simulink model "ac3_lat"  (Simulink 5.0)
settings: Solver=ode45  StartTime=0.0  StopTime=1000  RelTol=1e-3
values from neighbouring files (symbols this model uses):
  Dwash = [tau_w 1]    [ac3.m]
  JDa = [tau_a 1]    [ac3.m]
  JDr = [tau_r 1]    [ac3.m]
  JNa = [0 1]    [ac3.m]
  JNr = [0 1]    [ac3.m]
  Kphi = -30    [ac3.m]
  Nwash = [tau_w 0]    [ac3.m]
  rgain = (U0/g/tau_h)    (= 2.0039075773)    [ac3.m]
  theta0 = 0    [ac3.m]    (also in altit_simul.m; lecture4.m)
  U0 = 235.9    [ac3.m]    (also in altit_simul.m; lecture4.m = 774; newr.m)
libraries: aerolibanim x1, cstblocks x1
settings Model: LastModifiedBy=jonathan How

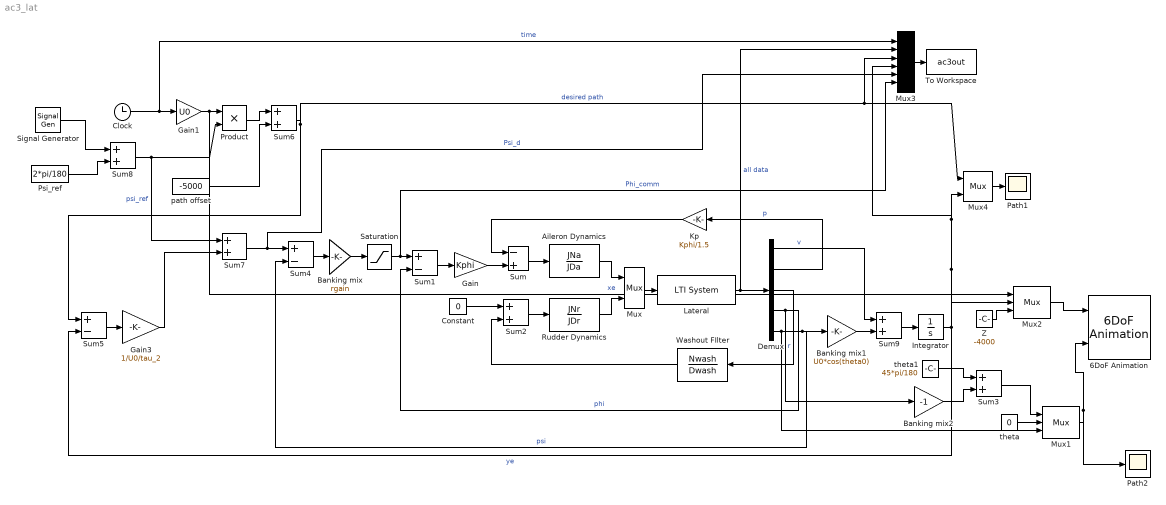
== system ac3_lat ==
  6DoF Animation : aerolibanim/6DoF Animation  u1=[0 4000 -6000 2000 -5000 -3000]  u2=0.1  u3=10  u4=[4000 0 -5000]  u5=Fly alongside  u6=[-100 0 -10]  u7=10  u8=on
  Aileron Dynamics : TransferFcn  Numerator=JNa  Denominator=JDa
  Banking mix : Gain  Gain=rgain  SaturateOnIntegerOverflow=on
  Banking mix1 : Gain  Gain=U0*cos(theta0)  SaturateOnIntegerOverflow=on
  Banking mix2 : Gain  Gain=-1  SaturateOnIntegerOverflow=on
  Clock : Clock
      settings: Decimation=10
  Constant : Constant  Value=0
  Demux : Demux  Outputs=5
  Gain : Gain  Gain=Kphi  SaturateOnIntegerOverflow=on
  Gain1 : Gain  Gain=U0  SaturateOnIntegerOverflow=on
  Gain3 : Gain  Gain=1/U0/tau_2  SaturateOnIntegerOverflow=on
  Integrator : Integrator
  Kp : Gain  Orientation=left  Gain=Kphi/1.5  SaturateOnIntegerOverflow=on
  Lateral : cstblocks/LTI System  sys=syslat2  IC=0
  Mux : Mux  Inputs=2
  Mux1 : Mux  Inputs=3
  Mux2 : Mux  Inputs=3
  Mux3 : Mux  Inputs=6
  Mux4 : Mux  Inputs=2
      settings: DisplayOption=signals
  Path1 : Scope
      settings: TimeRange=1000  YMin=-8000  YMax=9000
  Path2 : Scope
      settings: TimeRange=1000  YMin=-0.5  YMax=1.4
  Product : Product  SaturateOnIntegerOverflow=on  InputSameDT=on
  Psi_ref : Constant  Value=2*pi/180
  Rudder Dynamics : TransferFcn  Numerator=JNr  Denominator=JDr
  Saturation : Saturate  UpperLimit=30*pi/180  LowerLimit=-30*pi/180
  Signal Generator : SignalGenerator  WaveForm=square  Amplitude=3*pi/180  Frequency=.015  Units=rad/sec
  Sum : Sum  Inputs=-+  SaturateOnIntegerOverflow=on  InputSameDT=on
  Sum1 : Sum  Inputs=+-  SaturateOnIntegerOverflow=on  InputSameDT=on
  Sum{2..3,6..9} (6 alike) : Sum  SaturateOnIntegerOverflow=on  InputSameDT=on
  Sum4 : Sum  Inputs=+-  SaturateOnIntegerOverflow=on  InputSameDT=on
  Sum5 : Sum  Inputs=+-  SaturateOnIntegerOverflow=on  InputSameDT=on
  To Workspace : ToWorkspace  VariableName=ac3out  SampleTime=-1  SaveFormat=Array
  Washout FIlter : TransferFcn  Orientation=left  Numerator=Nwash  Denominator=Dwash
  Z : Constant  Value=-4000
  path offset : Constant  Value=-5000
  theta : Constant  Value=0
  theta1 : Constant  Value=45*pi/180
  wires:
  Aileron Dynamics/1 -> Mux/1
  Rudder Dynamics/1 -> Mux/2
  Mux/1 -> Lateral/1
  Lateral/1 -> Demux/1, Mux3/2  "all data"
  Demux/3 -> Washout FIlter/1  "r"
  Constant/1 -> Sum2/1
  Sum2/1 -> Rudder Dynamics/1
  Washout FIlter/1 -> Sum2/2
  Demux/2 -> Kp/1  "p"
  Kp/1 -> Sum/1
  Sum/1 -> Aileron Dynamics/1
  Demux/4 -> Sum1/2, Banking mix2/1  "phi"
  Sum1/1 -> Gain/1
  Demux/1 -> Sum9/1  "v"
  Demux/5 -> Sum4/2, Banking mix1/1, Mux1/3  "psi"
  Gain/1 -> Sum/2
  Sum4/1 -> Banking mix/1
  Banking mix/1 -> Saturation/1
  Product/1 -> Sum6/1
  Psi_ref/1 -> Sum8/2
  Signal Generator/1 -> Sum8/1
  Clock/1 -> Gain1/1, Mux3/1  "time"
  Gain1/1 -> Product/1, Mux2/1  "xe"
  path offset/1 -> Sum6/2
  Sum6/1 -> Sum5/1, Mux4/1, Mux3/3  "desired path"
  Sum8/1 -> Sum7/1, Product/2  "psi_ref"
  Sum7/1 -> Sum4/1, Mux3/5  "Psi_d"
  Sum5/1 -> Gain3/1
  Gain3/1 -> Sum7/2
  Banking mix1/1 -> Sum9/2
  Sum9/1 -> Integrator/1
  Integrator/1 -> Sum5/2, Mux4/2, Mux3/4, Mux2/2  "ye"
  Mux4/1 -> Path1/1
  Mux3/1 -> To Workspace/1
  Saturation/1 -> Sum1/1, Mux3/6  "Phi_comm"
  Mux1/1 -> 6DoF Animation/2, Path2/1
  Z/1 -> Mux2/3
  Mux2/1 -> 6DoF Animation/1
  theta/1 -> Mux1/2
  Banking mix2/1 -> Sum3/2
  theta1/1 -> Sum3/1
  Sum3/1 -> Mux1/1
